simulink model "Actuators_Dynamics"  (R2020a)
settings: Solver=FixedStepAuto  StartTime=0.0  StopTime=10.0  FixedStep=0.01  RelTol=1e-3
model workspace: external: MAT-File E:\Autopilot\Task 7\GP04_Task7_Codes\JETSTAR_FC4_Parameters.mat (data not in the file)
libraries: cstblocks x3
settings Model: Creator=mohan  LastModifiedBy=mohan

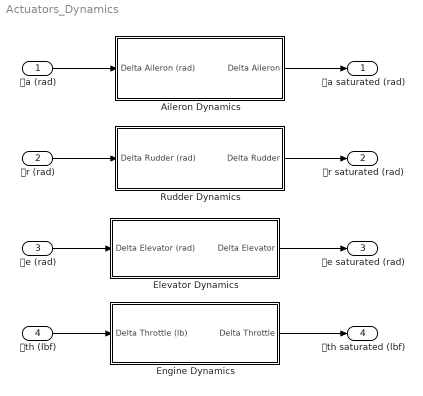
== system Actuators_Dynamics ==
  𝛿a (rad) : Inport
  𝛿r (rad) : Inport  Port=2
  𝛿e (rad) : Inport  Port=3
  𝛿th (lbf) : Inport  Port=4
  Aileron Dynamics : Subsystem  mask{delta_a_max=50}
      mask prompts: delta_a_max "Maximum Aileron Deflection (deg)"
      mask DialogControl ParameterGroupVar Prompt: Rudder Limits
  Elevator Dynamics : Subsystem  mask{delta_e_max=25}
      mask prompts: delta_e_max "Maximum Elevator Deflection (deg)"
      mask DialogControl ParameterGroupVar Prompt: Elevator Limits
  Engine Dynamics : Subsystem  mask{thrust_max=16000, thrust_min=-48000}
      mask prompts: thrust_max "Maximum Thrust"; thrust_min "Minimum Thrust"
      mask DialogControl ParameterGroupVar Prompt: Engine Limits
  Rudder Dynamics : Subsystem  mask{delta_r_max=25}
      mask prompts: delta_r_max "Maximum Rudder Deflection (deg)"
      mask DialogControl ParameterGroupVar Prompt: Rudder Limits
  𝛿a saturated (rad) : Outport
  𝛿r saturated (rad) : Outport  Port=2
  𝛿e saturated (rad) : Outport  Port=3
  𝛿th saturated (lbf) : Outport  Port=4
  wires:
  Aileron Dynamics/1(Delta Aileron) -> 𝛿a saturated (rad)/1
  𝛿a (rad)/1 -> Aileron Dynamics/1(Delta Aileron (rad))
  Rudder Dynamics/1(Delta Rudder) -> 𝛿r saturated (rad)/1
  𝛿r (rad)/1 -> Rudder Dynamics/1(Delta Rudder (rad))
  Elevator Dynamics/1(Delta Elevator) -> 𝛿e saturated (rad)/1
  𝛿e (rad)/1 -> Elevator Dynamics/1(Delta Elevator (rad))
  𝛿th (lbf)/1 -> Engine Dynamics/1(Delta Throttle (lb))
  Engine Dynamics/1(Delta Throttle) -> 𝛿th saturated (lbf)/1

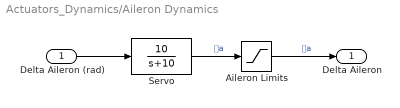
== system Actuators_Dynamics/Aileron Dynamics ==
  Delta Aileron (rad) : Inport
  Aileron Limits : Saturate  UpperLimit=delta_a_max*pi/180  LowerLimit=-delta_a_max*pi/180
  Servo : TransferFcn  Numerator=[10]  Denominator=[1 10]
  Delta Aileron : Outport
  wires:
  Servo/1 -> Aileron Limits/1  "𝛿a"
  Aileron Limits/1 -> Delta Aileron/1  "𝛿a"
  Delta Aileron (rad)/1 -> Servo/1

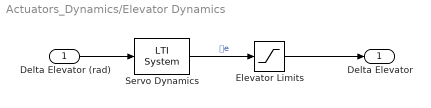
== system Actuators_Dynamics/Elevator Dynamics ==
  Delta Elevator (rad) : Inport
  Elevator Limits : Saturate  UpperLimit=delta_e_max*pi/180  LowerLimit=-delta_e_max*pi/180
  Servo Dynamics : cstblocks/LTI System  sys=-tf(10,[1 10])  IC=[]
  Delta Elevator : Outport
  wires:
  Servo Dynamics/1 -> Elevator Limits/1  "𝛿e"
  Elevator Limits/1 -> Delta Elevator/1
  Delta Elevator (rad)/1 -> Servo Dynamics/1

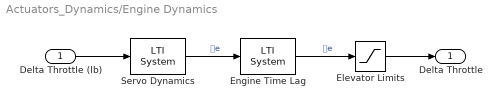
== system Actuators_Dynamics/Engine Dynamics ==
  Delta Throttle (lb) : Inport
  Elevator Limits : Saturate  UpperLimit=thrust_max  LowerLimit=thrust_min
  Engine Time Lag : cstblocks/LTI System  sys=tf(0.1,[1 0.1])  IC=[]
  Servo Dynamics : cstblocks/LTI System  sys=tf(10,[1 10])  IC=[]
  Delta Throttle : Outport
  wires:
  Servo Dynamics/1 -> Engine Time Lag/1  "𝛿e"
  Elevator Limits/1 -> Delta Throttle/1
  Delta Throttle (lb)/1 -> Servo Dynamics/1
  Engine Time Lag/1 -> Elevator Limits/1  "𝛿e"

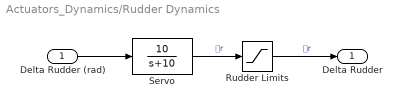
== system Actuators_Dynamics/Rudder Dynamics ==
  Delta Rudder (rad) : Inport
  Rudder Limits : Saturate  UpperLimit=delta_r_max*pi/180  LowerLimit=-delta_r_max*pi/180
  Servo : TransferFcn  Numerator=[10]  Denominator=[1 10]
  Delta Rudder : Outport
  wires:
  Servo/1 -> Rudder Limits/1  "𝛿r"
  Rudder Limits/1 -> Delta Rudder/1  "𝛿r"
  Delta Rudder (rad)/1 -> Servo/1
